simulink model "g_test"  (R2020a)
settings: Solver=VariableStepAuto  StartTime=0.0  StopTime=600  RelTol=1e-3
libraries: simulink x7, library_schuettgut x2
settings Model: Creator=Jonathan  LastModifiedBy=Jonathan

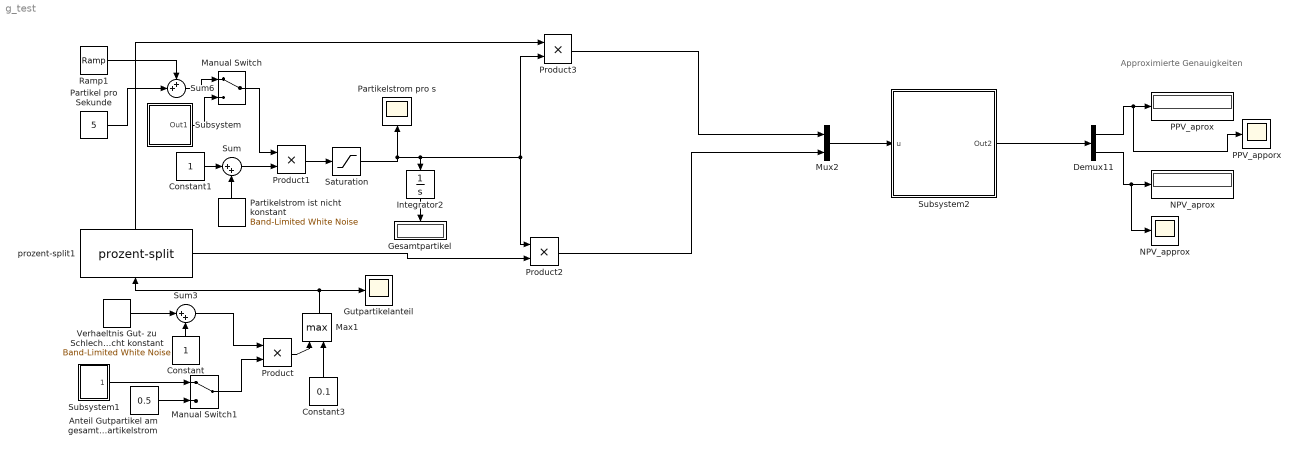
== system g_test ==
  note: Approximierte Genauigkeiten
  Anteil Gutpartikel am gesamten Partikelstrom : Constant  Value=0.5
  Constant : Constant
  Constant1 : Constant
  Constant3 : Constant  Value=0.1
  Demux11 : Demux  Outputs=2
  Gesamtpartikel : Display
  Gutpartikelanteil : Scope
  Integrator2 : Integrator
  Manual Switch : ManualSwitch
  Manual Switch1 : ManualSwitch
  Max1 : MinMax  Function=max  Inputs=2
  Mux2 : Mux  Inputs=2
  NPV_approx : Scope
  NPV_aprox : Display
  PPV_apporx : Scope
  PPV_aprox : Display
  Partikel pro Sekunde : Constant  Value=5
  Partikelstrom ist nicht konstant : simulink/Sources/Band-Limited White Noise  Cov=[0.00001]  Ts=0.1  seed=[23341]
  Partikelstrom pro s : Scope
  Product{,1..3} (4 alike) : Product
  Ramp1 : simulink/Sources/Ramp  slope=-0.01  start=200  InitialOutput=0
  Saturation : Saturate  UpperLimit=10  LowerLimit=0
  Subsystem : Subsystem
  Subsystem1 : Subsystem
  Subsystem2 : Subsystem
  Sum : Sum  Inputs=|++
  Sum3 : Sum  Inputs=|++
  Sum6 : Sum  Inputs=++|
  Verhaeltnis Gut- zu Schlechtpartikel ist nicht konstant : simulink/Sources/Band-Limited White Noise  Cov=[0.00001]  Ts=0.1  seed=[13341]
  prozent-split1 : library_schuettgut/prozent-split  SystemSampleTime=-1  Latency=0  AutoFrameSizeCalculation=off
      settings: PortSchema="{\"entries\":[{\"content\":{\"sides\":[{\"content\":{\"connectorIds\":[\"In1\"]},\"type\":\"ConnectorPlacement.EquallySpacedRectSide\",\"uuid\":\"ab8511c8-9f1d-48ad-bf24-85fd477f0bdd\"},{\"content\":{\"connectorIds\":[\"Out1\"],\"side\":\"RIGHT\"},\"type\":\"ConnectorPlacement.EquallySpacedRectSide\",\"uuid\":\"9ac1a19a-8176-444e-9f4d-7beffa0184e3\"},{\"content\":{\"connectorIds\":[\"Out2\"],\"side\":\"TOP\"},\"type\":\"ConnectorPlacement.EquallySpacedRectSide\",\"uuid\":\"376c2400-f821-4649-ab16-706a2da6117b\"}]},\"type\":\"ConnectorPlacement.EquallySpacedConnector\",\"uuid\":\"f6e72b2d-0467-4732-a018-d51f3a5db703\"}],\"packageUris\":[\"http://schema.mathworks.com/mf0/Connector/19700101\"],\"version\":\"1.0\"}"
  wires:
  Demux11/1 -> PPV_apporx/1, PPV_aprox/1
  Mux2/1 -> Subsystem2/1(u)
  Product3/1 -> Mux2/1
  Demux11/2 -> NPV_approx/1, NPV_aprox/1
  Subsystem2/1(Out2) -> Demux11/1
  Product2/1 -> Mux2/2
  Constant3/1 -> Max1/2
  Saturation/1 -> Product2/1, Product3/2, Integrator2/1, Partikelstrom pro s/1
  Ramp1/1 -> Sum6/1
  prozent-split1/1 -> Product3/1
  Subsystem/1(Out1) -> Manual Switch/2
  Partikel pro Sekunde/1 -> Sum6/2
  Verhaeltnis Gut- zu Schlechtpartikel ist nicht konstant/1 -> Sum3/1
  Sum6/1 -> Manual Switch/1
  prozent-split1/2 -> Product2/2
  Subsystem1/1(Out1) -> Manual Switch1/1
  Product1/1 -> Saturation/1
  Product/1 -> Max1/1
  Manual Switch1/1 -> Product/2
  Manual Switch/1 -> Product1/1
  Constant1/1 -> Sum/1
  Integrator2/1 -> Gesamtpartikel/1
  Partikelstrom ist nicht konstant/1 -> Sum/2
  Constant/1 -> Sum3/2
  Sum3/1 -> Product/1
  Anteil Gutpartikel am gesamten Partikelstrom/1 -> Manual Switch1/2
  Max1/1 -> prozent-split1/1, Gutpartikelanteil/1
  Sum/1 -> Product1/2

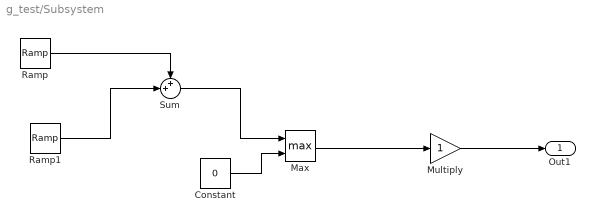
== system g_test/Subsystem ==
  Constant : Constant  Value=0
  Max : MinMax  Function=max  Inputs=2
  Multiply : Gain
  Ramp : simulink/Sources/Ramp  slope=10  start=0  InitialOutput=0
  Ramp1 : simulink/Sources/Ramp  slope=-20  start=100  InitialOutput=0
  Sum : Sum  Inputs=++|
  Out1 : Outport
  wires:
  Max/1 -> Multiply/1
  Constant/1 -> Max/2
  Sum/1 -> Max/1
  Ramp1/1 -> Sum/2
  Ramp/1 -> Sum/1
  Multiply/1 -> Out1/1

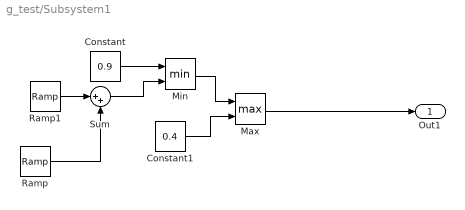
== system g_test/Subsystem1 ==
  Constant : Constant  Value=0.9
  Constant1 : Constant  Value=0.4
  Max : MinMax  Function=max  Inputs=2
  Min : MinMax  Inputs=2
  Ramp : simulink/Sources/Ramp  slope=0.01  start=20  InitialOutput=0.7
  Ramp1 : simulink/Sources/Ramp  slope=-0.03  start=150  InitialOutput=0
  Sum : Sum  Inputs=|++
  Out1 : Outport
  wires:
  Max/1 -> Out1/1
  Constant/1 -> Min/1
  Constant1/1 -> Max/2
  Min/1 -> Max/1
  Sum/1 -> Min/2
  Ramp1/1 -> Sum/1
  Ramp/1 -> Sum/2

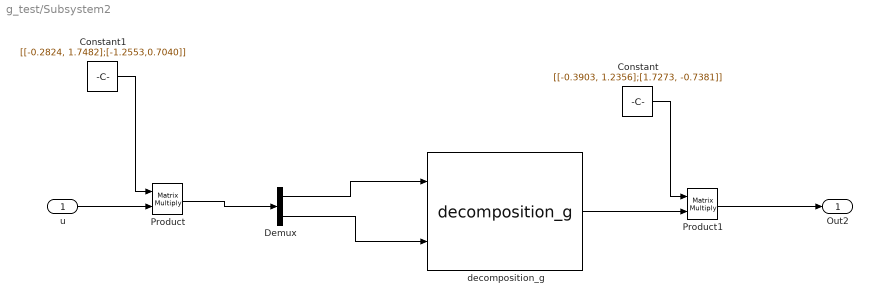
== system g_test/Subsystem2 ==
  u : Inport
  Constant : Constant  Value=[[-0.3903, 1.2356];[1.7273, -0.7381]]
  Constant1 : Constant  Value=[[-0.2824, 1.7482];[-1.2553,0.7040]]
  Demux : Demux  Outputs=2
  Product : Product  Multiplication=Matrix(*)
  Product1 : Product  Multiplication=Matrix(*)
  decomposition_g : library_schuettgut/decomposition_g  SystemSampleTime=-1  Latency=0  AutoFrameSizeCalculation=off
  Out2 : Outport
  wires:
  Product1/1 -> Out2/1
  Product/1 -> Demux/1
  Demux/1 -> decomposition_g/1
  Demux/2 -> decomposition_g/2
  decomposition_g/1 -> Product1/2
  u/1 -> Product/2
  Constant/1 -> Product1/1
  Constant1/1 -> Product/1
